simulink model "mult_signal"  (R2023a)
settings: Solver=FixedStepAuto  StartTime=0.0  StopTime=50.0  FixedStep=1e-5  RelTol=1e-3
model workspace (MAT data in the model file):
  sample = 0.05
undefined symbols (not defined in the file): LF
libraries: instrumentseriallib x3
settings Model: Creator=Aliso  LastModifiedBy=Aliso

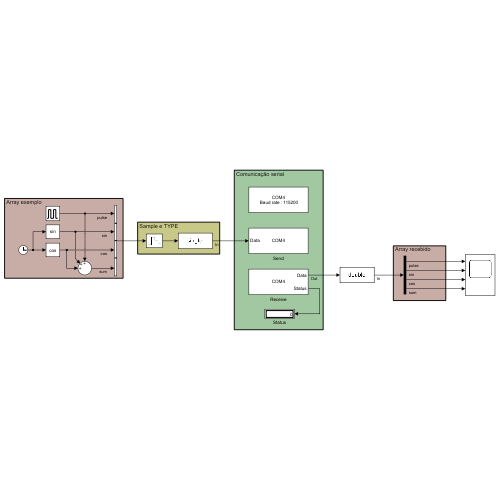
[thumbnail: Simulink's stored preview of the top-level diagram]
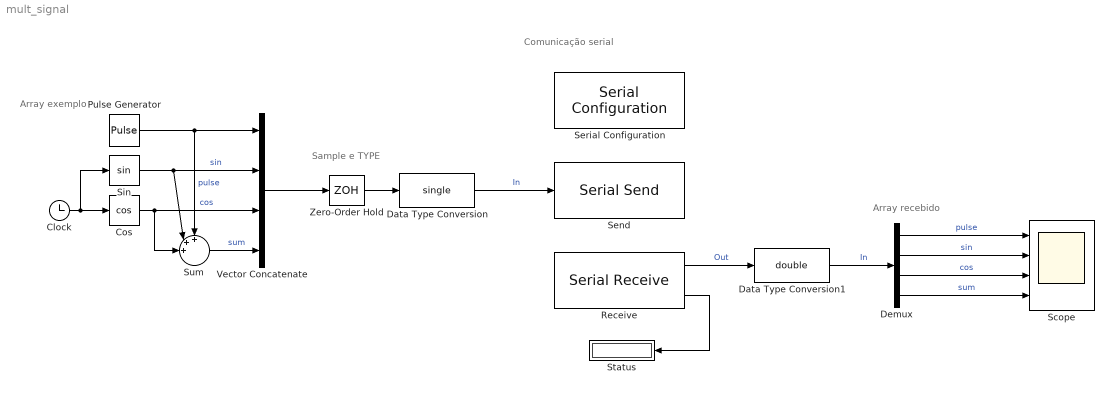
== system mult_signal ==
  note: Comunicação serial
  note: Array recebido
  note: Sample e TYPE
  note: Array exemplo
  Clock : Clock
  Cos : Trigonometry  Operator=cos
  Data Type Conversion : DataTypeConversion  OutDataTypeStr=single  SaturateOnIntegerOverflow=off  RndMeth=Floor  LockScale=on
  Data Type Conversion1 : DataTypeConversion  OutDataTypeStr=double  SaturateOnIntegerOverflow=off  RndMeth=Floor  LockScale=on
  Demux : Demux
  Pulse Generator : DiscretePulseGenerator  PulseType=Time based  Period=4  PulseWidth=50
  Receive : instrumentseriallib/Serial Receive  Priority=1  PortSel=COM4  Port=COM4  ComPort=COM4  DataType=single  SaveDataType=uint8  ToggleHeader=on  Header=[65]  ToggleTerminator=on  Terminator=LF ('\n')  CustomTerminator=[]  InputFormat=Column major  ToggleDataSize=on  DataSize=[1 4]  EnableBlockingMode=off  ActionDataUnavailable=Output last received value  ActionWhenDataUnavailable=Output last received value  CustomValue=0  SampleTime=sample/2  SimulateUsing=Interpreted execution  BlockInModel=on  aMode=1
      settings: LibrarySourceBlock=c2000lib/Host Communication/Serial Receive
  Scope : Scope  NumInputPorts=4
  Send : instrumentseriallib/Serial Send  Priority=1  PortSel=COM4  Port=COM4  ComPort=COM4  Header=[65]  Terminator=LF ('\n')  CustomTerminator=[]  EnableBlockingMode=on  SimulateUsing=Interpreted execution  BlockInModel=on  aMode=1
      settings: LibrarySourceBlock=c2000lib/Host Communication/Serial Send
  Serial Configuration : instrumentseriallib/Serial Configuration  Priority=-200000  PortSel=COM4  Port=COM4  ComPort=COM4  BaudRate=115200  DataBits=8  Parity=none  StopBits=1  ByteOrder=little-endian  FlowControl=none  Timeout=10  SimulateUsing=Interpreted execution  BlockInModel=on  aMode=1
      settings: LibrarySourceBlock=c2000lib/Host Communication/Serial Configuration
  Sin : Trigonometry
  Status : Display
  Sum : Sum  Inputs=+++||
  Vector Concatenate : Concatenate  NumInputs=4
  Zero-Order Hold : ZeroOrderHold  SampleTime=sample
  wires:
  Vector Concatenate/1 -> Zero-Order Hold/1
  Zero-Order Hold/1 -> Data Type Conversion/1
  Demux/1 -> Scope/1  "pulse"
  Demux/2 -> Scope/2  "sin"
  Demux/3 -> Scope/3  "cos"
  Demux/4 -> Scope/4  "sum"
  Receive/2 -> Status/1
  Data Type Conversion/1 -> Send/1  "In"
  Pulse Generator/1 -> Sum/1, Vector Concatenate/1  "pulse"
  Sin/1 -> Vector Concatenate/2, Sum/2  "sin"
  Cos/1 -> Sum/3, Vector Concatenate/3  "cos"
  Clock/1 -> Sin/1, Cos/1
  Receive/1 -> Data Type Conversion1/1  "Out"
  Data Type Conversion1/1 -> Demux/1  "In"
  Sum/1 -> Vector Concatenate/4  "sum"
